simulink model "DatosSignals"  (Simulink 7.9)
settings: Solver=ode45  StartTime=0.0  StopTime=10.0  RelTol=1e-8  AbsTol=1e-8
libraries: simulink x1
settings Model: Creator=estudiantes  LastModifiedBy=estudiantes
settings OptimizationCC: InitFltsAndDblsToZero=on
settings DebuggingCC: SaveWithParameterizedLinksMsg=none  SignalResolutionControl=TryResolveAllWithWarning  MultiTaskDSMMsg=warning  MultiTaskCondExecSysMsg=none  FcnCallInpInsideContextMsg=Use local settings  StrictBusMsg=Warning
settings RTWCC: IncludeERTFirstTime=on
settings GRTTargetCC: TargetFcnLib=ansi_tfl_tmw.mat  CombineOutputUpdateFcns=off  GRTInterface=on

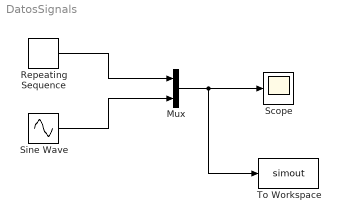
== system DatosSignals ==
  Mux : Mux  Inputs=2
  Repeating Sequence : simulink/Sources/Repeating Sequence  rep_seq_t=[0 1 2 3 4]  rep_seq_y=[0 1 0 -1 0]
  Scope : Scope
  Sine Wave : Sin  Frequency=2*pi/4  SampleTime=0
  To Workspace : ToWorkspace  VariableName=simout  SampleTime=0.01
  wires:
  Repeating Sequence/1 -> Mux/1
  Sine Wave/1 -> Mux/2
  Mux/1 -> Scope/1, To Workspace/1
